simulink model "simulink_transducer"  (R2025a)
settings: Solver=VariableStepAuto  StartTime=0.0  StopTime=10  RelTol=1e-3
libraries: spsSeriesRLCBranchLib x38, spsImpedanceMeasurementLib x6, sps_lib x1
settings Model: Creator=ASUS  LastModifiedBy=ASUS

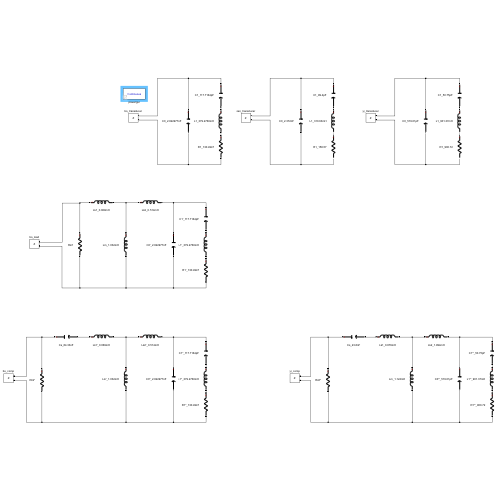
[thumbnail: Simulink's stored preview of the top-level diagram]
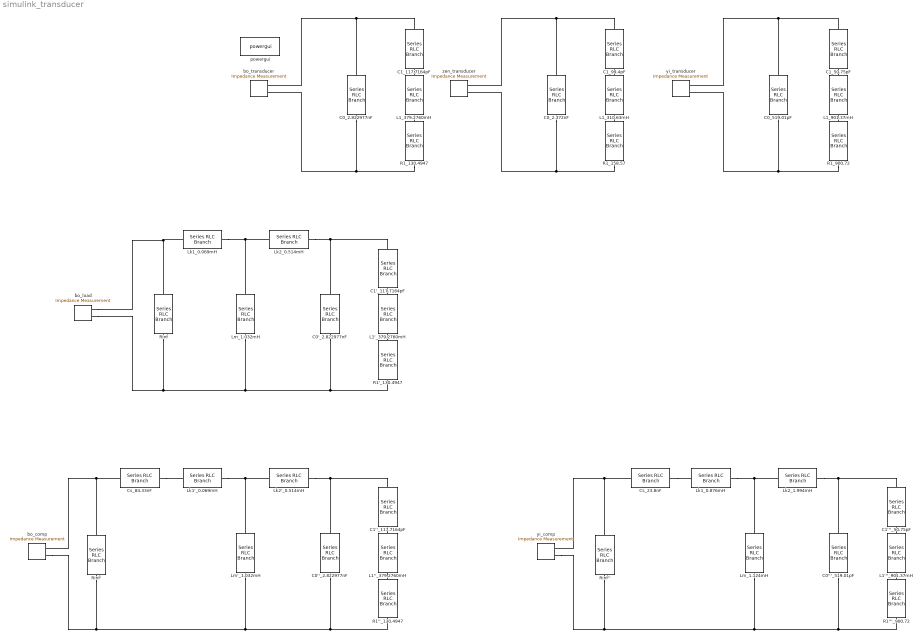
== system simulink_transducer ==
  C0'''_519.01pF : spsSeriesRLCBranchLib/Series RLC Branch  LConnTagsString=__new0  RConnTagsString=__new0  BranchType=C  Resistance=0  Inductance=1e-3  SetiL0=off  InitialCurrent=0  Capacitance=519.01e-12  Setx0=off  InitialVoltage=0  Measurements=None
  C0''_2.822977nF : spsSeriesRLCBranchLib/Series RLC Branch  LConnTagsString=__new0  RConnTagsString=__new0  BranchType=C  Resistance=0  Inductance=1e-3  SetiL0=off  InitialCurrent=0  Capacitance=2.822977e-9  Setx0=off  InitialVoltage=0  Measurements=None
  C0'_2.822977nF : spsSeriesRLCBranchLib/Series RLC Branch  LConnTagsString=__new0  RConnTagsString=__new0  BranchType=C  Resistance=0  Inductance=1e-3  SetiL0=off  InitialCurrent=0  Capacitance=2.822977e-9  Setx0=off  InitialVoltage=0  Measurements=None
  C0_2.372nF : spsSeriesRLCBranchLib/Series RLC Branch  LConnTagsString=__new0  RConnTagsString=__new0  BranchType=C  Resistance=0  Inductance=1e-3  SetiL0=off  InitialCurrent=0  Capacitance=2.372e-9  Setx0=off  InitialVoltage=0  Measurements=None
  C0_2.822977nF : spsSeriesRLCBranchLib/Series RLC Branch  LConnTagsString=__new0  RConnTagsString=__new0  BranchType=C  Resistance=0  Inductance=1e-3  SetiL0=off  InitialCurrent=0  Capacitance=2.822977e-9  Setx0=off  InitialVoltage=0  Measurements=None
  C0_519.01pF : spsSeriesRLCBranchLib/Series RLC Branch  LConnTagsString=__new0  RConnTagsString=__new0  BranchType=C  Resistance=0  Inductance=1e-3  SetiL0=off  InitialCurrent=0  Capacitance=519.01e-12  Setx0=off  InitialVoltage=0  Measurements=None
  C1'''_50.75pF : spsSeriesRLCBranchLib/Series RLC Branch  LConnTagsString=__new0  RConnTagsString=__new0  BranchType=C  Resistance=0  Inductance=1e-3  SetiL0=off  InitialCurrent=0  Capacitance=50.75e-12  Setx0=off  InitialVoltage=0  Measurements=None
  C1''_117.7164pF : spsSeriesRLCBranchLib/Series RLC Branch  LConnTagsString=__new0  RConnTagsString=__new0  BranchType=C  Resistance=0  Inductance=1e-3  SetiL0=off  InitialCurrent=0  Capacitance=117.7164e-12  Setx0=off  InitialVoltage=0  Measurements=None
  C1'_117.7164pF : spsSeriesRLCBranchLib/Series RLC Branch  LConnTagsString=__new0  RConnTagsString=__new0  BranchType=C  Resistance=0  Inductance=1e-3  SetiL0=off  InitialCurrent=0  Capacitance=117.7164e-12  Setx0=off  InitialVoltage=0  Measurements=None
  C1_117.7164pF : spsSeriesRLCBranchLib/Series RLC Branch  LConnTagsString=__new0  RConnTagsString=__new0  BranchType=C  Resistance=0  Inductance=1e-3  SetiL0=off  InitialCurrent=0  Capacitance=117.7164e-12  Setx0=off  InitialVoltage=0  Measurements=None
  C1_50.75pF : spsSeriesRLCBranchLib/Series RLC Branch  LConnTagsString=__new0  RConnTagsString=__new0  BranchType=C  Resistance=0  Inductance=1e-3  SetiL0=off  InitialCurrent=0  Capacitance=50.75e-12  Setx0=off  InitialVoltage=0  Measurements=None
  C1_99.4pF : spsSeriesRLCBranchLib/Series RLC Branch  LConnTagsString=__new0  RConnTagsString=__new0  BranchType=C  Resistance=0  Inductance=1e-3  SetiL0=off  InitialCurrent=0  Capacitance=99.4e-12  Setx0=off  InitialVoltage=0  Measurements=None
  Cs_23.8nF : spsSeriesRLCBranchLib/Series RLC Branch  LConnTagsString=__new0  RConnTagsString=__new0  BranchType=C  Resistance=0  Inductance=1e-3  SetiL0=off  InitialCurrent=0  Capacitance=23.8e-9  Setx0=off  InitialVoltage=0  Measurements=None
  Cs_84.33nF : spsSeriesRLCBranchLib/Series RLC Branch  LConnTagsString=__new0  RConnTagsString=__new0  BranchType=C  Resistance=0  Inductance=1e-3  SetiL0=off  InitialCurrent=0  Capacitance=30e-9  Setx0=off  InitialVoltage=0  Measurements=None
  L1'''_901.37mH : spsSeriesRLCBranchLib/Series RLC Branch  LConnTagsString=__new0  RConnTagsString=__new0  BranchType=L  Resistance=0  Inductance=901.37e-3  SetiL0=off  InitialCurrent=0  Capacitance=0  Setx0=off  InitialVoltage=0  Measurements=None
  L1''_379.2760mH : spsSeriesRLCBranchLib/Series RLC Branch  LConnTagsString=__new0  RConnTagsString=__new0  BranchType=L  Resistance=0  Inductance=379.2760e-3  SetiL0=off  InitialCurrent=0  Capacitance=0  Setx0=off  InitialVoltage=0  Measurements=None
  L1'_379.2760mH : spsSeriesRLCBranchLib/Series RLC Branch  LConnTagsString=__new0  RConnTagsString=__new0  BranchType=L  Resistance=0  Inductance=379.2760e-3  SetiL0=off  InitialCurrent=0  Capacitance=0  Setx0=off  InitialVoltage=0  Measurements=None
  L1_310.63mH : spsSeriesRLCBranchLib/Series RLC Branch  LConnTagsString=__new0  RConnTagsString=__new0  BranchType=L  Resistance=0  Inductance=310.63e-3  SetiL0=off  InitialCurrent=0  Capacitance=0  Setx0=off  InitialVoltage=0  Measurements=None
  L1_379.2760mH : spsSeriesRLCBranchLib/Series RLC Branch  LConnTagsString=__new0  RConnTagsString=__new0  BranchType=L  Resistance=0  Inductance=379.2760e-3  SetiL0=off  InitialCurrent=0  Capacitance=0  Setx0=off  InitialVoltage=0  Measurements=None
  L1_901.37mH : spsSeriesRLCBranchLib/Series RLC Branch  LConnTagsString=__new0  RConnTagsString=__new0  BranchType=L  Resistance=0  Inductance=901.37e-3  SetiL0=off  InitialCurrent=0  Capacitance=0  Setx0=off  InitialVoltage=0  Measurements=None
  Lk1'_0.069mH : spsSeriesRLCBranchLib/Series RLC Branch  LConnTagsString=__new0  RConnTagsString=__new0  BranchType=L  Resistance=0  Inductance=0.069e-3  SetiL0=off  InitialCurrent=0  Capacitance=0  Setx0=off  InitialVoltage=0  Measurements=None
  Lk1_0.069mH : spsSeriesRLCBranchLib/Series RLC Branch  LConnTagsString=__new0  RConnTagsString=__new0  BranchType=L  Resistance=0  Inductance=0.069e-3  SetiL0=off  InitialCurrent=0  Capacitance=0  Setx0=off  InitialVoltage=0  Measurements=None
  Lk1_0.876mH : spsSeriesRLCBranchLib/Series RLC Branch  LConnTagsString=__new0  RConnTagsString=__new0  BranchType=L  Resistance=0  Inductance=0.876e-3  SetiL0=off  InitialCurrent=0  Capacitance=0  Setx0=off  InitialVoltage=0  Measurements=None
  Lk2'_0.514mH : spsSeriesRLCBranchLib/Series RLC Branch  LConnTagsString=__new0  RConnTagsString=__new0  BranchType=L  Resistance=0  Inductance=0.514e-3  SetiL0=off  InitialCurrent=0  Capacitance=0  Setx0=off  InitialVoltage=0  Measurements=None
  Lk2_0.514mH : spsSeriesRLCBranchLib/Series RLC Branch  LConnTagsString=__new0  RConnTagsString=__new0  BranchType=L  Resistance=0  Inductance=0.514e-3  SetiL0=off  InitialCurrent=0  Capacitance=0  Setx0=off  InitialVoltage=0  Measurements=None
  Lk2_1.994mH : spsSeriesRLCBranchLib/Series RLC Branch  LConnTagsString=__new0  RConnTagsString=__new0  BranchType=L  Resistance=0  Inductance=1.994e-3  SetiL0=off  InitialCurrent=0  Capacitance=0  Setx0=off  InitialVoltage=0  Measurements=None
  Lm'_1.032mH : spsSeriesRLCBranchLib/Series RLC Branch  LConnTagsString=__new0  RConnTagsString=__new0  BranchType=L  Resistance=0  Inductance=1.032e-3  SetiL0=off  InitialCurrent=0  Capacitance=0  Setx0=off  InitialVoltage=0  Measurements=None
  Lm_1.032mH : spsSeriesRLCBranchLib/Series RLC Branch  LConnTagsString=__new0  RConnTagsString=__new0  BranchType=L  Resistance=0  Inductance=1.032e-3  SetiL0=off  InitialCurrent=0  Capacitance=0  Setx0=off  InitialVoltage=0  Measurements=None
  Lm_1.124mH : spsSeriesRLCBranchLib/Series RLC Branch  LConnTagsString=__new0  RConnTagsString=__new0  BranchType=L  Resistance=0  Inductance=1.124e-3  SetiL0=off  InitialCurrent=0  Capacitance=0  Setx0=off  InitialVoltage=0  Measurements=None
  R1'''_900.72 : spsSeriesRLCBranchLib/Series RLC Branch  LConnTagsString=__new0  RConnTagsString=__new0  BranchType=R  Resistance=900.72  Inductance=1e-3  SetiL0=off  InitialCurrent=0  Capacitance=0  Setx0=off  InitialVoltage=0  Measurements=None
  R1''_130.4947 : spsSeriesRLCBranchLib/Series RLC Branch  LConnTagsString=__new0  RConnTagsString=__new0  BranchType=R  Resistance=130.4947  Inductance=1e-3  SetiL0=off  InitialCurrent=0  Capacitance=0  Setx0=off  InitialVoltage=0  Measurements=None
  R1'_130.4947 : spsSeriesRLCBranchLib/Series RLC Branch  LConnTagsString=__new0  RConnTagsString=__new0  BranchType=R  Resistance=130.4947  Inductance=1e-3  SetiL0=off  InitialCurrent=0  Capacitance=0  Setx0=off  InitialVoltage=0  Measurements=None
  R1_130.4947 : spsSeriesRLCBranchLib/Series RLC Branch  LConnTagsString=__new0  RConnTagsString=__new0  BranchType=R  Resistance=130.4947  Inductance=1e-3  SetiL0=off  InitialCurrent=0  Capacitance=0  Setx0=off  InitialVoltage=0  Measurements=None
  R1_158.57 : spsSeriesRLCBranchLib/Series RLC Branch  LConnTagsString=__new0  RConnTagsString=__new0  BranchType=R  Resistance=158.57  Inductance=1e-3  SetiL0=off  InitialCurrent=0  Capacitance=0  Setx0=off  InitialVoltage=0  Measurements=None
  R1_900.72 : spsSeriesRLCBranchLib/Series RLC Branch  LConnTagsString=__new0  RConnTagsString=__new0  BranchType=R  Resistance=900.72  Inductance=1e-3  SetiL0=off  InitialCurrent=0  Capacitance=0  Setx0=off  InitialVoltage=0  Measurements=None
  Rinf : spsSeriesRLCBranchLib/Series RLC Branch  LConnTagsString=__new0  RConnTagsString=__new0  BranchType=R  Resistance=10000000  Inductance=1e-3  SetiL0=off  InitialCurrent=0  Capacitance=0  Setx0=off  InitialVoltage=0  Measurements=None
  Rinf' : spsSeriesRLCBranchLib/Series RLC Branch  LConnTagsString=__new0  RConnTagsString=__new0  BranchType=R  Resistance=10000000  Inductance=1e-3  SetiL0=off  InitialCurrent=0  Capacitance=0  Setx0=off  InitialVoltage=0  Measurements=None
  Rinf'' : spsSeriesRLCBranchLib/Series RLC Branch  LConnTagsString=__new0  RConnTagsString=__new0  BranchType=R  Resistance=10000000  Inductance=1e-3  SetiL0=off  InitialCurrent=0  Capacitance=0  Setx0=off  InitialVoltage=0  Measurements=None
  bo_comp : spsImpedanceMeasurementLib/Impedance Measurement  LConnTagsString=+|-  Factor=1
      settings: LibrarySourceBlock=sps_lib/Sensors and Measurements/Impedance Measurement
  bo_load : spsImpedanceMeasurementLib/Impedance Measurement  LConnTagsString=+|-  Factor=1
      settings: LibrarySourceBlock=sps_lib/Sensors and Measurements/Impedance Measurement
  bo_transducer : spsImpedanceMeasurementLib/Impedance Measurement  LConnTagsString=+|-  Factor=1
      settings: LibrarySourceBlock=sps_lib/Sensors and Measurements/Impedance Measurement
  powergui : sps_lib/powergui  Priority=1  SimulationMode=Continuous  SampleTime=50e-6  frequency=60  Iterations=50  frequencyindice=60  Pbase=100e6  ErrMax=1e-4  UnitsV=kV  UnitsW=MW  buscounter=0  FunctionMessages=off  echomessages=off  EnableUseOfTLC=off  CurrentSourceSwitches=off  DisableSnubberDevices=off  DisableRonSwitches=off  DisableVfSwitches=off  DisplayEquations=off  AutomaticDiscreteSolvers=off  SolverType=Tustin/Backward Euler (TBE)  Interpol=off  ExternalGateDelay=off  methode=off  Ts=100  x0status=blocks  SPID=on  SwTol=0  HookPort=off  NonlinearTolerance=1e-4  nMaxIteration=100  ContinueOnMaxIteration=off  RestoreLinks=warning  ResistiveCurrentMeasurement=off  Frange=[0:2:500]  Ylog=off  Xlog=on  ShowGrid=off  save=off  variable=ZData  structure=0  ZoomFFT=off  StartTime=0.0  cycles=1  DisplayStyle=1  fundamental=60  FreqAxis=off  MaxFrequency=1000  frequencyindicesteady=1  RmsSteady=1  display=off
  yi_comp : spsImpedanceMeasurementLib/Impedance Measurement  LConnTagsString=+|-  Factor=1
      settings: LibrarySourceBlock=sps_lib/Sensors and Measurements/Impedance Measurement
  yi_transducer : spsImpedanceMeasurementLib/Impedance Measurement  LConnTagsString=+|-  Factor=1
      settings: LibrarySourceBlock=sps_lib/Sensors and Measurements/Impedance Measurement
  zen_transducer : spsImpedanceMeasurementLib/Impedance Measurement  LConnTagsString=+|-  Factor=1
      settings: LibrarySourceBlock=sps_lib/Sensors and Measurements/Impedance Measurement
  connections:
  C1_99.4pF/RConn1 -- L1_310.63mH/LConn1
  R1_158.57/LConn1 -- L1_310.63mH/RConn1
  C0_2.372nF/LConn1 -- C1_99.4pF/LConn1 -- zen_transducer/LConn1
  R1_158.57/RConn1 -- C0_2.372nF/RConn1 -- zen_transducer/LConn2
  bo_transducer/LConn1 -- C0_2.822977nF/LConn1 -- C1_117.7164pF/LConn1
  bo_transducer/LConn2 -- R1_130.4947/RConn1 -- C0_2.822977nF/RConn1
  C1_117.7164pF/RConn1 -- L1_379.2760mH/LConn1
  R1_130.4947/LConn1 -- L1_379.2760mH/RConn1
  C0'_2.822977nF/LConn1 -- C1'_117.7164pF/LConn1 -- Lk2_0.514mH/RConn1
  C0'_2.822977nF/RConn1 -- bo_load/LConn2 -- Rinf/RConn1 -- Lm_1.032mH/RConn1 -- R1'_130.4947/RConn1
  R1'_130.4947/LConn1 -- L1'_379.2760mH/RConn1
  C1'_117.7164pF/RConn1 -- L1'_379.2760mH/LConn1
  Lm_1.032mH/LConn1 -- Lk1_0.069mH/RConn1 -- Lk2_0.514mH/LConn1
  bo_load/LConn1 -- Lk1_0.069mH/LConn1 -- Rinf/LConn1
  C0''_2.822977nF/RConn1 -- Lm'_1.032mH/RConn1 -- Rinf'/RConn1 -- bo_comp/LConn2 -- R1''_130.4947/RConn1
  C0''_2.822977nF/LConn1 -- Lk2'_0.514mH/RConn1 -- C1''_117.7164pF/LConn1
  Lm'_1.032mH/LConn1 -- Lk1'_0.069mH/RConn1 -- Lk2'_0.514mH/LConn1
  R1''_130.4947/LConn1 -- L1''_379.2760mH/RConn1
  C1''_117.7164pF/RConn1 -- L1''_379.2760mH/LConn1
  yi_comp/LConn2 -- Rinf''/RConn1 -- Lm_1.124mH/RConn1 -- C0'''_519.01pF/RConn1 -- R1'''_900.72/RConn1
  Lm_1.124mH/LConn1 -- Lk1_0.876mH/RConn1 -- Lk2_1.994mH/LConn1
  C0'''_519.01pF/LConn1 -- Lk2_1.994mH/RConn1 -- C1'''_50.75pF/LConn1
  C1'''_50.75pF/RConn1 -- L1'''_901.37mH/LConn1
  R1'''_900.72/LConn1 -- L1'''_901.37mH/RConn1
  Rinf'/LConn1 -- Cs_84.33nF/LConn1 -- bo_comp/LConn1
  Cs_84.33nF/RConn1 -- Lk1'_0.069mH/LConn1
  yi_transducer/LConn1 -- C0_519.01pF/LConn1 -- C1_50.75pF/LConn1
  yi_transducer/LConn2 -- C0_519.01pF/RConn1 -- R1_900.72/RConn1
  R1_900.72/LConn1 -- L1_901.37mH/RConn1
  C1_50.75pF/RConn1 -- L1_901.37mH/LConn1
  Rinf''/LConn1 -- Cs_23.8nF/LConn1 -- yi_comp/LConn1
  Cs_23.8nF/RConn1 -- Lk1_0.876mH/LConn1
